simulink model "sim_5_2 - Copy"  (R2017b)
settings: Solver=VariableStepAuto  StartTime=0.0  StopTime=10.0  RelTol=1e-3
settings Model: Creator=nadav  LastModifiedBy=nadav

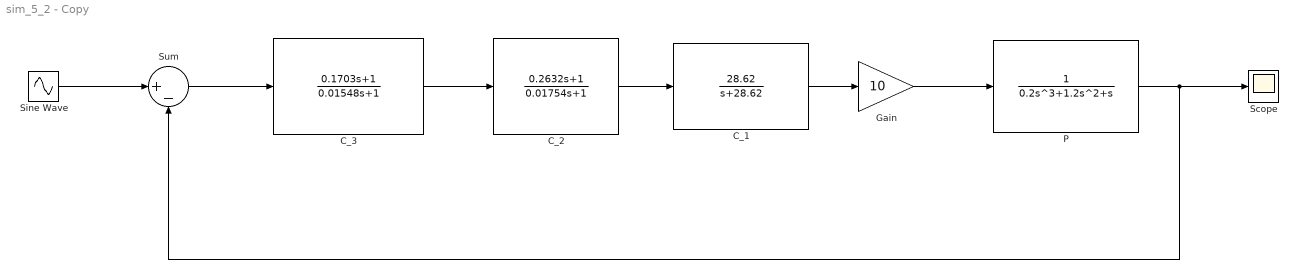
== system sim_5_2 - Copy ==
  C_1 : TransferFcn  Numerator=[28.62]  Denominator=[1 28.62]
  "C_2 " : TransferFcn  Numerator=[0.2632 1]  Denominator=[0.01754 1]
  C_3 : TransferFcn  Numerator=[0.1703 1]  Denominator=[0.01548 1]
  Gain : Gain  Gain=10
  "P " : TransferFcn  Denominator=[0.2 1.2 1 0]
  Scope : Scope
  Sine Wave : Sin  Amplitude=2  Frequency=17.5  SampleTime=0
  Sum : Sum  Inputs=|+-
  wires:
  Sine Wave/1 -> Sum/1
  Gain/1 -> "P "/1
  C_1/1 -> Gain/1
  "C_2 "/1 -> C_1/1
  C_3/1 -> "C_2 "/1
  Sum/1 -> C_3/1
  "P "/1 -> Scope/1, Sum/2
